simulink model "BLOC_Driver1"  (R2016a)
settings: Solver=FixedStepAuto  StartTime=0.0  StopTime=10.0  FixedStep=hev_dt  RelTol=1e-3
undefined symbols (not defined in the file): dri_ki, dri_kp, hev_dt
libraries: simulink x6, simulink_extras x1
settings Model: Creator=Florent  LastModifiedBy=Florent
settings OptimizationCC: DefaultParameterBehavior=Inlined  OptimizeModelRefInitCode=on  LifeSpan=1
settings RTWCC: SystemTargetFile=ert.tlc  TemplateMakefile=ert_default_tmf  GenerateReport=on  IncludeHyperlinkInReport=on  LaunchReport=on  TargetLang=C++  GenerateTraceInfo=on  GenerateTraceReport=on  GenerateTraceReportSl=on  GenerateTraceReportSf=on  GenerateTraceReportEml=on
settings CodeAppCC: ForceParamTrailComments=on  OperatorAnnotations=on  SimulinkDataObjDesc=on  SFDataObjDesc=on  MATLABFcnDesc=on  InsertBlockDesc=on  MATLABSourceComments=on
settings ERTTargetCC: GenerateSampleERTMain=on  MultiInstanceERTCode=on  CodeInterfacePackaging=C++ class  InlinedParameterPlacement=NonHierarchical  RootIOFormat=Structure reference  ERTCustomFileTemplate=example_file_process.tlc

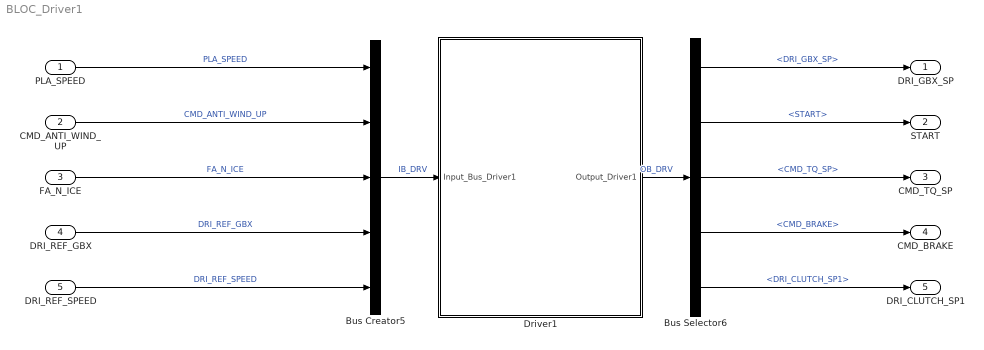
== system BLOC_Driver1 ==
  PLA_SPEED : Inport
  CMD_ANTI_WIND_UP : Inport  Port=2
  FA_N_ICE : Inport  Port=3
  DRI_REF_GBX : Inport  Port=4  SampleTime=hev_dt
  DRI_REF_SPEED : Inport  Port=5
  Bus Creator5 : BusCreator  Inputs=5
  Bus Selector6 : BusSelector  OutputSignals=DRI_GBX_SP,START,CMD_TQ_SP,CMD_BRAKE,DRI_CLUTCH_SP1
  Driver1 : Subsystem  TreatAsAtomicUnit=on
  DRI_GBX_SP : Outport
  START : Outport  Port=2
  CMD_TQ_SP : Outport  Port=3
  CMD_BRAKE : Outport  Port=4
  DRI_CLUTCH_SP1 : Outport  Port=5
  wires:
  DRI_REF_SPEED/1 -> Bus Creator5/5  "DRI_REF_SPEED"
  DRI_REF_GBX/1 -> Bus Creator5/4  "DRI_REF_GBX"
  PLA_SPEED/1 -> Bus Creator5/1  "PLA_SPEED"
  CMD_ANTI_WIND_UP/1 -> Bus Creator5/2  "CMD_ANTI_WIND_UP"
  FA_N_ICE/1 -> Bus Creator5/3  "FA_N_ICE"
  Bus Creator5/1 -> Driver1/1(Input_Bus_Driver1)  "IB_DRV"
  Driver1/1(Output_Driver1) -> Bus Selector6/1  "OB_DRV"
  Bus Selector6/1 -> DRI_GBX_SP/1  "<DRI_GBX_SP>"
  Bus Selector6/2 -> START/1  "<START>"
  Bus Selector6/3 -> CMD_TQ_SP/1  "<CMD_TQ_SP>"
  Bus Selector6/4 -> CMD_BRAKE/1  "<CMD_BRAKE>"
  Bus Selector6/5 -> DRI_CLUTCH_SP1/1  "<DRI_CLUTCH_SP1>"

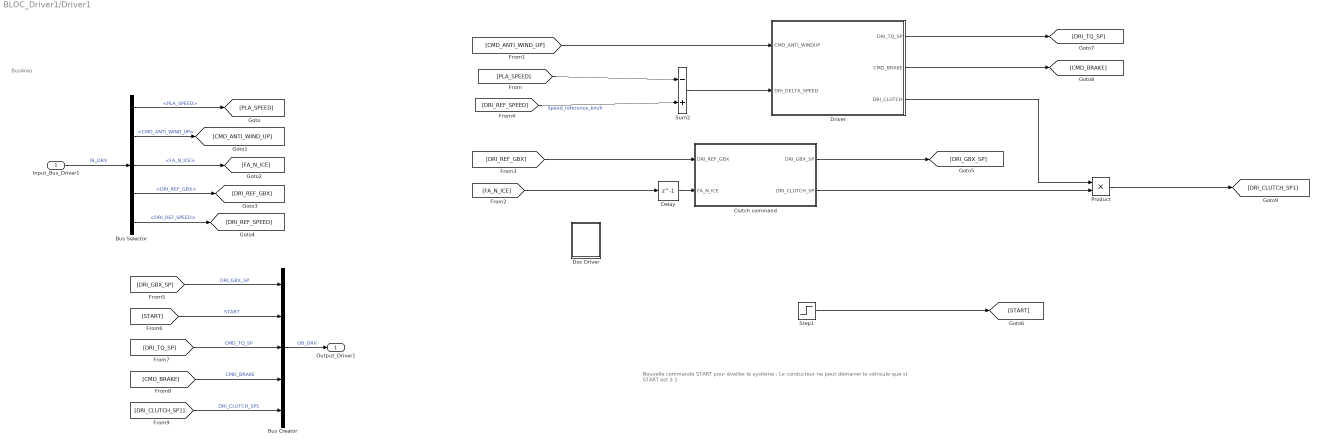
== system BLOC_Driver1/Driver1 ==
  note: BusArea
  note: Nouvelle commande START pour éveiller le système : Le conducteur ne peut démarrer le véhicule que si START est à 1
  Input_Bus_Driver1 : Inport
  Bus Creator : BusCreator  Inputs=5
  Bus Selector : BusSelector  OutputSignals=PLA_SPEED,CMD_ANTI_WIND_UP,FA_N_ICE,DRI_REF_GBX,DRI_REF_SPEED
  Clutch command : Subsystem
  Delay : Delay  DelayLength=1
  Doc Driver : Subsystem
      settings: OpenFcn=open('Documents\Driver.pdf')
      mask Display: fprintf('DOC')
  Driver : Subsystem
  Product : Product
  Step1 : Step  Time=0  SampleTime=0
  Sum2 : Sum  Inputs=-|+  SampleTime=hev_dt
  Output_Driver1 : Outport
  wires:
  [CMD_ANTI_WIND_UP] -> Driver/1(CMD_ANTI_WINDUP)
  [DRI_REF_GBX] -> Clutch command/1(DRI_REF_GBX)
  [DRI_REF_SPEED] -> Sum2/2  "Speed_reference_km/h"
  Driver/1(DRI_TQ_SP) -> [DRI_TQ_SP]
  Driver/2(CMD_BRAKE) -> [CMD_BRAKE]
  Sum2/1 -> Driver/2(DRI_DELTA_SPEED)
  [PLA_SPEED] -> Sum2/1
  Step1/1 -> [START]
  [FA_N_ICE] -> Delay/1
  Clutch command/1(DRI_GBX_SP) -> [DRI_GBX_SP]
  Clutch command/2(DRI_CLUTCH_SP) -> Product/2
  Delay/1 -> Clutch command/2(FA_N_ICE)
  Driver/3(DRI_CLUTCH) -> Product/1
  Product/1 -> [DRI_CLUTCH_SP1]
  Input_Bus_Driver1/1 -> Bus Selector/1  "IB_DRV"
  Bus Selector/1 -> [PLA_SPEED]  "<PLA_SPEED>"
  Bus Selector/2 -> [CMD_ANTI_WIND_UP]  "<CMD_ANTI_WIND_UP>"
  Bus Selector/3 -> [FA_N_ICE]  "<FA_N_ICE>"
  Bus Selector/4 -> [DRI_REF_GBX]  "<DRI_REF_GBX>"
  Bus Selector/5 -> [DRI_REF_SPEED]  "<DRI_REF_SPEED>"
  Bus Creator/1 -> Output_Driver1/1  "OB_DRV"
  [DRI_GBX_SP] -> Bus Creator/1  "DRI_GBX_SP"
  [START] -> Bus Creator/2  "START"
  [DRI_TQ_SP] -> Bus Creator/3  "CMD_TQ_SP"
  [CMD_BRAKE] -> Bus Creator/4  "CMD_BRAKE"
  [DRI_CLUTCH_SP1] -> Bus Creator/5  "DRI_CLUTCH_SP1"

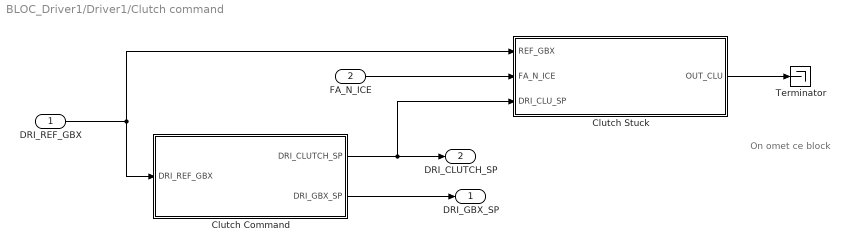
== system BLOC_Driver1/Driver1/Clutch command ==
  note: On omet ce block
  DRI_REF_GBX : Inport
  FA_N_ICE : Inport  Port=2
  Clutch Command : Subsystem
  Clutch Stuck : Subsystem
  Terminator : Terminator
  DRI_GBX_SP : Outport
  DRI_CLUTCH_SP : Outport  Port=2
  wires:
  DRI_REF_GBX/1 -> Clutch Command/1(DRI_REF_GBX), Clutch Stuck/1(REF_GBX)
  Clutch Command/2(DRI_GBX_SP) -> DRI_GBX_SP/1
  FA_N_ICE/1 -> Clutch Stuck/2(FA_N_ICE)
  Clutch Command/1(DRI_CLUTCH_SP) -> DRI_CLUTCH_SP/1, Clutch Stuck/3(DRI_CLU_SP)
  Clutch Stuck/1(OUT_CLU) -> Terminator/1

== system BLOC_Driver1/Driver1/Doc Driver ==

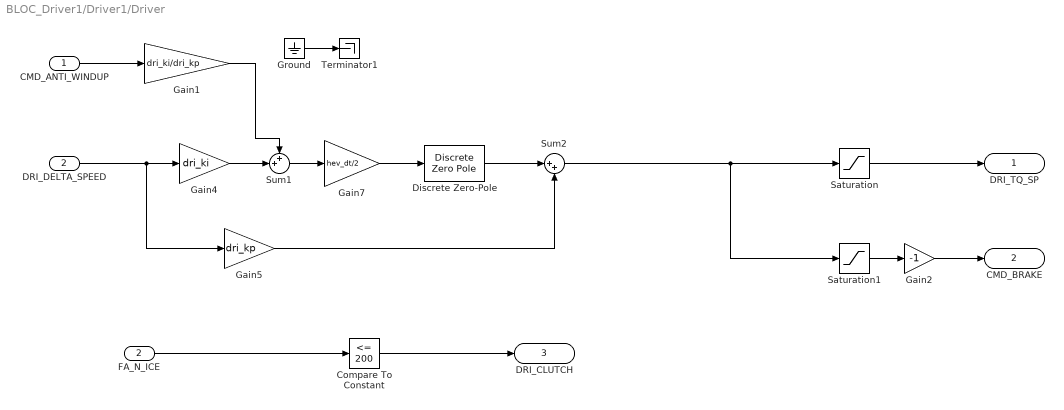
== system BLOC_Driver1/Driver1/Driver ==
  CMD_ANTI_WINDUP : Inport
  DRI_DELTA_SPEED : Inport  Port=2
  Compare To Constant : simulink/Logic and Bit Operations/Compare To Constant  relop=<=  const=200  OutDataTypeStr=uint8
  Discrete Zero-Pole : DiscreteZeroPole  Zeros=[-1]  Poles=[1]  Gain=1  SampleTime=hev_dt
  FA_N_ICE : InportShadow  Port=2
  Gain1 : Gain  Gain=dri_ki/dri_kp  SampleTime=hev_dt
  Gain2 : Gain  Gain=-1
  Gain4 : Gain  Gain=dri_ki  SampleTime=hev_dt
  Gain5 : Gain  Gain=dri_kp  SampleTime=hev_dt
  Gain7 : Gain  Gain=hev_dt/2  SampleTime=hev_dt
  Ground : Ground
  Saturation : Saturate  UpperLimit=inf  LowerLimit=0
  Saturation1 : Saturate  UpperLimit=0  LowerLimit=-inf
  Sum1 : Sum  Inputs=++|  SampleTime=hev_dt
  Sum2 : Sum  Inputs=|++  SampleTime=hev_dt
  Terminator1 : Terminator
  DRI_TQ_SP : Outport
  CMD_BRAKE : Outport  Port=2
  DRI_CLUTCH : Outport  Port=3
  wires:
  Gain5/1 -> Sum2/2
  Gain4/1 -> Sum1/2
  Sum1/1 -> Gain7/1
  Discrete Zero-Pole/1 -> Sum2/1
  CMD_ANTI_WINDUP/1 -> Gain1/1
  DRI_DELTA_SPEED/1 -> Gain5/1, Gain4/1
  Sum2/1 -> Saturation1/1, Saturation/1
  Gain7/1 -> Discrete Zero-Pole/1
  Saturation/1 -> DRI_TQ_SP/1
  Saturation1/1 -> Gain2/1
  Ground/1 -> Terminator1/1
  Gain1/1 -> Sum1/1
  Gain2/1 -> CMD_BRAKE/1
  FA_N_ICE/1 -> Compare To Constant/1
  Compare To Constant/1 -> DRI_CLUTCH/1

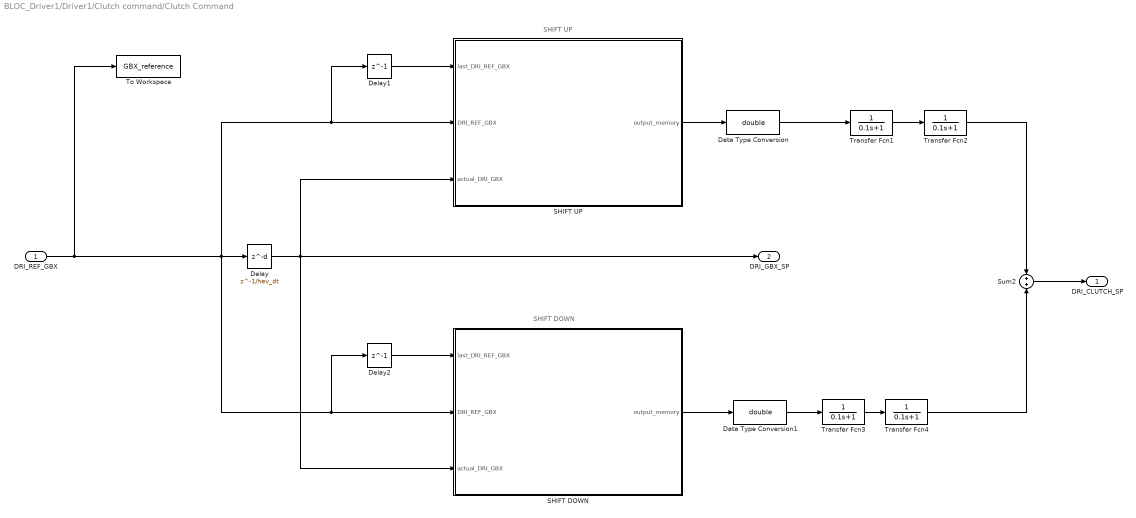
== system BLOC_Driver1/Driver1/Clutch command/Clutch Command ==
  note: SHIFT DOWN
  note: SHIFT UP
  DRI_REF_GBX : Inport
  Data Type Conversion : DataTypeConversion  OutDataTypeStr=double
  Data Type Conversion1 : DataTypeConversion  OutDataTypeStr=double
  Delay : Delay  DelayLength=1/hev_dt  SampleTime=hev_dt
  Delay1 : Delay  DelayLength=1
  Delay2 : Delay  DelayLength=1
  SHIFT DOWN : Stateflow chart  TreatAsAtomicUnit=on
  SHIFT UP : Stateflow chart  TreatAsAtomicUnit=on
  Sum2 : Sum
  To Workspace : ToWorkspace  VariableName=GBX_reference  SampleTime=-1
  Transfer Fcn{1..4} (4 alike) : TransferFcn  Denominator=[0.1 1]
  DRI_CLUTCH_SP : Outport
  DRI_GBX_SP : Outport  Port=2
  wires:
  SHIFT UP/1(output_memory) -> Data Type Conversion/1
  Sum2/1 -> DRI_CLUTCH_SP/1
  SHIFT DOWN/1(output_memory) -> Data Type Conversion1/1
  Delay2/1 -> SHIFT DOWN/1(last_DRI_REF_GBX)
  DRI_REF_GBX/1 -> SHIFT UP/2(DRI_REF_GBX), Delay1/1, Delay/1, SHIFT DOWN/2(DRI_REF_GBX), Delay2/1, To Workspace/1
  Delay/1 -> SHIFT UP/3(actual_DRI_GBX), DRI_GBX_SP/1, SHIFT DOWN/3(actual_DRI_GBX)
  Delay1/1 -> SHIFT UP/1(last_DRI_REF_GBX)
  Transfer Fcn1/1 -> Transfer Fcn2/1
  Transfer Fcn3/1 -> Transfer Fcn4/1
  Data Type Conversion1/1 -> Transfer Fcn3/1
  Transfer Fcn2/1 -> Sum2/1
  Transfer Fcn4/1 -> Sum2/2
  Data Type Conversion/1 -> Transfer Fcn1/1

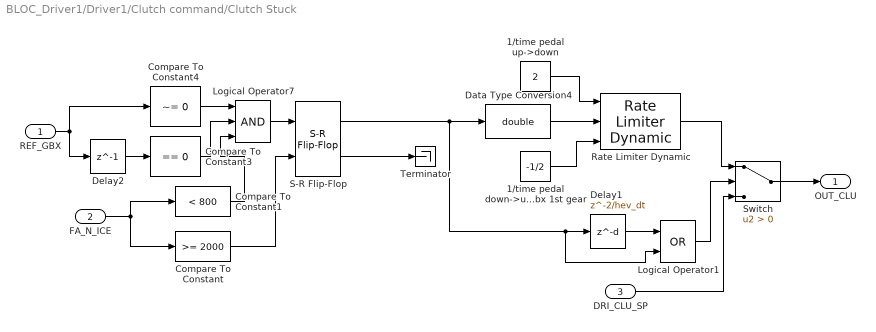
== system BLOC_Driver1/Driver1/Clutch command/Clutch Stuck ==
  REF_GBX : Inport
  FA_N_ICE : Inport  Port=2
  DRI_CLU_SP : Inport  Port=3
  1/time pedal down->up  gbx 1st gear : Constant  Value=-1/2
  1/time pedal up->down : Constant  Value=2
  Compare To Constant : simulink/Logic and Bit Operations/Compare To Constant  relop=>=  const=2000  OutDataTypeStr=boolean
  Compare To Constant1 : simulink/Logic and Bit Operations/Compare To Constant  relop=<  const=800  OutDataTypeStr=boolean
  Compare To Constant3 : simulink/Logic and Bit Operations/Compare To Constant  relop===  const=0  OutDataTypeStr=uint8
  Compare To Constant4 : simulink/Logic and Bit Operations/Compare To Constant  relop=~=  const=0  OutDataTypeStr=uint8
  Data Type Conversion4 : DataTypeConversion  OutDataTypeStr=double  SampleTime=hev_dt
  Delay1 : Delay  DelayLength=2/hev_dt  SampleTime=hev_dt
  Delay2 : Delay  DelayLength=1  SampleTime=hev_dt
  Logical Operator1 : Logic  Operator=OR  AllPortsSameDT=off  OutDataTypeStr=boolean  SampleTime=hev_dt
  Logical Operator7 : Logic  Inputs=3  AllPortsSameDT=off  OutDataTypeStr=boolean  SampleTime=hev_dt
  Rate Limiter Dynamic : simulink/Discontinuities/Rate Limiter Dynamic
  S-R Flip-Flop : simulink_extras/Flip Flops/S-R Flip-Flop  initial_condition=0
  Switch : Switch  Criteria=u2 > Threshold
  Terminator : Terminator
  OUT_CLU : Outport
  wires:
  REF_GBX/1 -> Delay2/1, Compare To Constant4/1
  S-R Flip-Flop/2 -> Terminator/1
  Compare To Constant/1 -> S-R Flip-Flop/2
  Rate Limiter Dynamic/1 -> Switch/1
  S-R Flip-Flop/1 -> Logical Operator1/2, Delay1/1, Data Type Conversion4/1
  Compare To Constant4/1 -> Logical Operator7/1
  Delay2/1 -> Compare To Constant3/1
  Compare To Constant3/1 -> Logical Operator7/2
  FA_N_ICE/1 -> Compare To Constant/1, Compare To Constant1/1
  Delay1/1 -> Logical Operator1/1
  Data Type Conversion4/1 -> Rate Limiter Dynamic/2
  1/time pedal up->down/1 -> Rate Limiter Dynamic/1
  Compare To Constant1/1 -> Logical Operator7/3
  Logical Operator1/1 -> Switch/2
  Logical Operator7/1 -> S-R Flip-Flop/1
  1/time pedal down->up  gbx 1st gear/1 -> Rate Limiter Dynamic/3
  Switch/1 -> OUT_CLU/1
  DRI_CLU_SP/1 -> Switch/3

== stateflow chart BLOC_Driver1/Driver1/Clutch command/Clutch Command/SHIFT DOWN ==
  state First_state
    entry: output_memory = 1;
  state Second_state
    entry: output_memory = 0;
  (default) -> (junction 11)
  (junction 11) -> First_state [order 1] : [last_DRI_REF_GBX > DRI_REF_GBX]
  (junction 11) -> Second_state [order 2] : [DRI_REF_GBX == actual_DRI_GBX]
  First_state -> Second_state : [DRI_REF_GBX == actual_DRI_GBX]
  Second_state -> First_state : [last_DRI_REF_GBX > DRI_REF_GBX]
  data: output_memory output; last_DRI_REF_GBX input; DRI_REF_GBX input; actual_DRI_GBX input

== stateflow chart BLOC_Driver1/Driver1/Clutch command/Clutch Command/SHIFT UP ==
  state First_state
    entry: output_memory = 1;
  state Second_state
    entry: output_memory = 0;
  (default) -> (junction 11)
  (junction 11) -> First_state [order 1] : [last_DRI_REF_GBX < DRI_REF_GBX]
  (junction 11) -> Second_state [order 2] : [DRI_REF_GBX == actual_DRI_GBX]
  First_state -> Second_state : [DRI_REF_GBX == actual_DRI_GBX]
  Second_state -> First_state : [last_DRI_REF_GBX < DRI_REF_GBX]
  data: output_memory output; last_DRI_REF_GBX input; DRI_REF_GBX input; actual_DRI_GBX input
